simulink model "manipulator_cl"  (R2018b)
settings: Solver=ode45  StartTime=0.0  StopTime=4  RelTol=1e-6
values from neighbouring files (symbols this model uses):
  sys_titop = directDynamicsSuper*tf(1, [1 0])    [titopSimple_model.m]    (also in titop_model.m)
undefined symbols (not defined in the file or in its folder): alpha_rel, kp1, kp2, kv1, Kv2, rad_deg
settings Model: Creator=a.brugnoli  LastModifiedBy=a.brugnoli

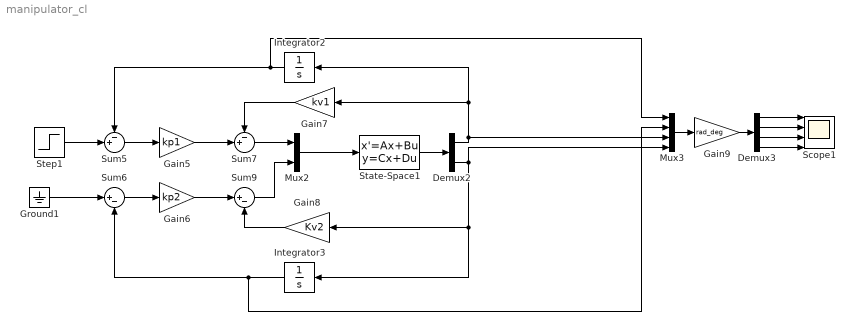
== system manipulator_cl ==
  Demux2 : Demux  Outputs=2
  Demux3 : Demux
  Gain5 : Gain  Gain=kp1
  Gain6 : Gain  Gain=kp2
  Gain7 : Gain  Gain=kv1
  Gain8 : Gain  Gain=Kv2
  Gain9 : Gain  Gain=rad_deg
  Ground1 : Ground
  Integrator2 : Integrator
  Integrator3 : Integrator
  Mux2 : Mux  Inputs=2
  Mux3 : Mux
  Scope1 : Scope  NumInputPorts=4
  State-Space1 : StateSpace  A=sys_titop.A  B=sys_titop.B  C=sys_titop.C  D=sys_titop.D  InitialCondition=0
  Step1 : Step  After=alpha_rel  SampleTime=0
  Sum5 : Sum  Inputs=-+|
  Sum6 : Sum  Inputs=|+-
  Sum7 : Sum  Inputs=-+|
  Sum9 : Sum  Inputs=|+-
  wires:
  Demux3/1 -> Scope1/1
  Gain8/1 -> Sum9/2
  Sum9/1 -> Mux2/2
  Gain5/1 -> Sum7/2
  Step1/1 -> Sum5/2
  Gain7/1 -> Sum7/1
  Demux3/4 -> Scope1/4
  Gain6/1 -> Sum9/1
  Ground1/1 -> Sum6/1
  Demux2/1 -> Gain7/1, Integrator2/1, Mux3/3
  State-Space1/1 -> Demux2/1
  Sum7/1 -> Mux2/1
  Mux2/1 -> State-Space1/1
  Integrator2/1 -> Mux3/1, Sum5/1
  Gain9/1 -> Demux3/1
  Mux3/1 -> Gain9/1
  Integrator3/1 -> Mux3/2, Sum6/2
  Demux3/3 -> Scope1/3
  Sum5/1 -> Gain5/1
  Demux3/2 -> Scope1/2
  Sum6/1 -> Gain6/1
  Demux2/2 -> Integrator3/1, Gain8/1, Mux3/4
